simulink library "dspbdsp2"  (Simulink 3.00)
values from neighbouring files (symbols this model uses):
  b = tmp(end-3:end)    [aboutdspblks.m]    (also in dspcsum.m = find_system(blk,'LookUnderMasks','all', 'FollowLinks','on', )
libraries: simulink3 x5, dspbdsp2 x2, dspvect2 x2, dspddes2 x1, dspmtrx2 x1, dsplinalg x1
settings Model: Creator=szlotkin  LastModifiedBy=sconahan

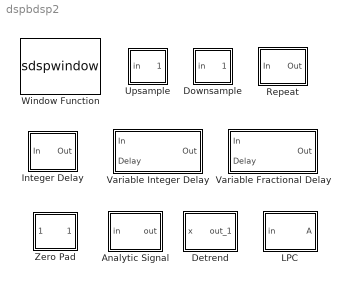
== system dspbdsp2 ==
  Analytic Signal : Subsystem  mask(Analytic Signal){N=100, frame=off, numChans=1}
      mask prompts: N "Filter order (must be even):"; frame "Frame-Based Inputs:"; numChans "Number of Channels"
      mask help: Complex analytic signal of input.
      mask init:
      | [x,y] = dspblkanalytic('icon');
      mask Help: web(dspbhelp);
      mask CallbackString: |dspblkanalytic|
      mask Display: plot(x,y)
  Detrend : Subsystem
      mask Type: Detrend
      mask Description: Remove linear trend from vector input.
      mask Help: web(dspbhelp);
      mask Display: plot(0,0,100,100,[12 20 24 32 38 44 49 54 67 69 71 78 81 89],[56 76 60 79 75 83 80 87 65 76 84 86 91 89],[],[],[],[],[],[],[12 20 24 32 38 44 49 54 67 69 71 78 81 89],[12 31 13 31 27 34 30 36 13 23 30 31 34 32],[4 96],[61 90],[47 47 42 47 52],[64 44 50 44 50],[4 96],[23 23])
  Downsample : Subsystem  mask(Downsample){N=2, phase=0, ic=0, sample_mode=off, frame=off, nchans=1, mode=Maintain input frame size}
      mask prompts: N "Downsample factor, N:"; phase "Sample offset (0 to N-1):"; ic "Initial condition:"; sample_mode "Enforce single-rate"; frame "Frame-based inputs"; nchans "Number of channels:"; mode "Framing:"
      mask help: Downsample by an integer factor. Optional sample offset must be an integer in range (0, N-1).
      mask init:
      | [s,x,y] = dspblkdsamp('icon',N, &1);
      mask Help: web(dspbhelp);
      mask StyleString: edit,edit,edit,checkbox,checkbox,edit,popup(Maintain input frame size|Maintain input frame rate)
      mask CallbackString: ||||dspblkdsamp||
      mask Display:
      | plot(x,y);
      | text(.6,.4,s);
  Integer Delay : Subsystem  mask(Integer Delay){delay=1, ic=0, frame=off, df=on, numChans=1}
      mask prompts: delay "Delay in samples:"; ic "Initial Conditions:"; frame "Frame-Based Inputs"; df "Direct Feedthrough (deselect only if delay >= frame size)"; numChans "Number of Channels:"
      mask help:
      | Delay discrete-time input by a fixed integer number of sample periods.
      |
      | In frame-based mode, feedback loops can be made computable by deselecting "Direct Feedthrough".  This is valid only if the minimum delay value is at least as large as the frame size.
      mask init:
      | str = ['-' &1];
      | dx = 0.01*length(str);
      | if strcmp(frame,'off'), numChans=-1; end
      | delay=double(delay);
      mask Help: web(dspbhelp);
      mask CallbackString: ||dspblkdly||
      mask Display: text(0.42-dx, 0.4, 'z'); text(0.5-dx, 0.6, str);
  LPC : Subsystem  mask(LPC){ord=-1}
      mask prompts: ord "Prediction order (-1 for length(u)-1):"
      mask help: Output the coefficients of an Nth order forward linear predictor such that the sum of the squares of the errors is minimized.
      mask init:
      | if ord==-1,
      |    pad = -1; acf=-1;
      | else
      |    pad = ord+1; acf=ord;
      | end
      mask Help: web(dspbhelp);
      mask Display: disp('LPC')
  Repeat : Subsystem  mask(Repeat){N=5, ic=0, frame=off, nchans=1, mode=Maintain input frame size}
      mask prompts: N "Repetition count:"; ic "Initial conditions:"; frame "Frame-based inputs"; nchans "Number of channels:"; mode "Framing:"
      mask help: Repeat input samples N times.
      mask init:
      | s = dspblkrepeat('icon',N, &1);
      mask Help: web(dspbhelp);
      mask StyleString: edit,edit,checkbox,edit,popup(Maintain input frame size|Maintain input frame rate)
      mask CallbackString: ||dspblkrepeat||
      mask Display: disp(s);
  Upsample : Subsystem  mask(Upsample){N=3, phase=0, ic=0, frame=off, nchans=1, mode=Maintain input frame size}
      mask prompts: N "Upsample factor, N:"; phase "Sample offset (0 to N-1):"; ic "Initial condition:"; frame "Frame-based inputs"; nchans "Number of channels:"; mode "Framing:"
      mask help: Upsample by inserting N-1 zeros between input samples. Optional sample offset must be an integer in range (0, N-1).
      mask init:
      | [s,x,y] = dspblkupsamp('icon',N, &1);
      mask Help: web(dspbhelp);
      mask StyleString: edit,edit,edit,checkbox,edit,popup(Maintain input frame size|Maintain input frame rate)
      mask CallbackString: |||dspblkupsamp||
      mask Display:
      | plot(x,y)
      | text(.6,.4,s);
  Variable Fractional Delay : Subsystem  mask(Variable Fractional Delay){mode=Linear Interpolation, dmax=100, L=4, R=10, alpha=0.5, ic=0, frame=off, numChans=1}
      mask prompts: dmax "Maximum delay in samples:"; L "Interpolation filter half-length:"; R "Interpolation points per input sample:"; alpha "Normalized input bandwidth (0 to 1):"; ic "Initial Conditions:"; frame "Frame-Based Inputs"; numChans "Number of Channels:"
      mask help: Delay discrete-time input by a time-varying fractional number of sample periods, as specified by the "delay" input. Delay must be a real vector signal with one delay value per frame element. The FIR filter is designed using "intfilt" from the Signal Processing Toolbox.
      mask init:
      | [b,str] = dspblkvfdly(mode,R,L,alpha);
      | if strcmp(frame,'off'), numChans=-1; end
      mask Help: web(dspbhelp);
      mask StyleString: popup(Linear Interpolation|FIR Interpolation),edit,edit,edit,edit,edit,checkbox,edit
      mask CallbackString: dspblkvfdly||||||dspblkvfdly|
      mask Display:
      | text(0.5,0.4,'z','horiz','right')
      | text(0.5,0.6,'-f','horiz','left')
  Variable Integer Delay : Subsystem  mask(Variable Integer Delay){dmax=100, ic=0, frame=off, numChans=1}
      mask prompts: dmax "Maximum delay in samples:"; ic "Initial Conditions:"; frame "Frame-Based Inputs"; numChans "Number of Channels:"
      mask help: Delay discrete-time input by a time-varying integer number of sample periods specified by the "delay" input. Delay is a real vector signal with one delay value per sample period. For frame-based operation, the delay input can have one delay per sample period or one delay per frame.
      mask init:
      | str = dspblkvidly(1);
      | if strcmp(frame,'off'), numChans=-1; end
      mask Help: web(dspbhelp);
      mask CallbackString: ||dspblkvidly|
      mask Display:
      | text(0.5,0.4,'z','horiz','right')
      | text(0.5,0.6,'-i','horiz','left')
  Window Function : S-Function  FunctionName=sdspwindow  Parameters=winmode,wintype,N,Rs,beta,winsamp,NChans  PortCounts=[]  SFunctionModules=''  mask(Window Function){winmode=Apply window to input, wintype=Hamming, N=64, Rs=50, beta=10, winsamp=Symmetric, NChans=1}
      mask prompts: winmode "Operation:"; wintype "Window Type:"; N "Window length:"; Rs "Stopband attenuation in dB:"; winsamp "Sampling:"; NChans "Number of channels:"
      mask help: Generate window function and apply to input vector.
      mask init:
      | [x,y,str,ports] = dspblkwinfcn('icon',Rs,beta);
      mask Help: web(dspbhelp);
      mask StyleString: popup(Apply window to input|Generate window|Generate and apply window),popup(Bartlett|Blackman|Boxcar|Chebyshev|Hamming|Hann|Hanning|Kaiser|Triang),edit,edit,edit,popup(Symmetric|Periodic),edit
      mask CallbackString: dspblkwinfcn|dspblkwinfcn|||||
      mask Display:
      | plot(x,y); text(.2,.85,str);
      | port_label(ports(1).type,ports(1).port,ports(1).txt);
      | port_label(ports(2).type,ports(2).port,ports(2).txt);
      | port_label(ports(3).type,ports(3).port,ports(3).txt);
  Zero Pad : Subsystem  mask(Zero Pad){pad=-1, trunc=on, nchans=1}
      mask prompts: pad "Output frame size (-1 to inherit input size):"; trunc "Allow truncation of input"; nchans "Number of channels:"
      mask help: Pad input frame with zeros.
      mask Help: web(dspbhelp);
      mask Display: plot(0,0,100,100,[51 44 44 51],[92 92 8 8],[73 80 80 73],[92 92 8 8],[56 68],[80 80],[56 68],[72 72],[56 68],[64 64],[56 68],[56 56],[56 68],[48 48],[56 68],[40 40],[64 60 56 55 56 60 64 68 69 68 64],[32 32 28 22 16 12 12 16 22 28 32],[24 24 40 36 40 36],[52 24 24 28 24 20])

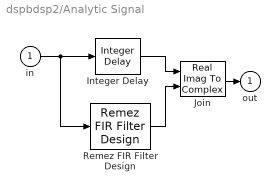
== system dspbdsp2/Analytic Signal ==
  in : Inport  Port=1  PortWidth=-1  SampleTime=-1  DataType=auto
      settings: SignalType=auto
  Integer Delay : dspbdsp2/Integer Delay  delay=N/2  ic=0  frame=off  df=on  numChans=1
  Join : RealImagToComplex  Input=RealAndImag  ConstantPart=0
  Remez FIR Filter Design : dspddes2/Remez FIR Filter Design  filttype=Hilbert Transform  F=[0.05 .95]  A=[1 1]  W=1  N=N  frame=off  numCHANS=1
  out : Outport  Port=1  InitialOutput=0
  wires:
  in/1 -> Remez FIR Filter Design/1, Integer Delay/1
  Join/1 -> out/1
  Integer Delay/1 -> Join/1
  Remez FIR Filter Design/1 -> Join/2

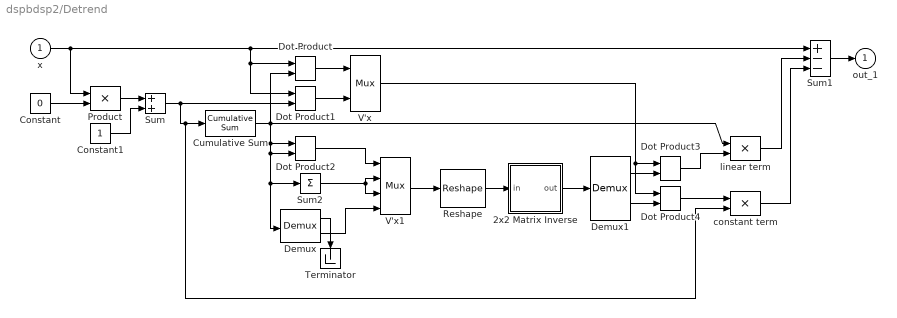
== system dspbdsp2/Detrend ==
  x : Inport  Port=1  PortWidth=-1  SampleTime=-1  DataType=auto
      settings: SignalType=auto
  2x2 Matrix Inverse : Subsystem
      mask Type: Invert 2x2 Matrix
      mask Display: disp('Invert\n2x2')
  Constant : Constant  Value=0
  Constant1 : Constant  Value=1
  Cumulative Sum : dspvect2/Cumulative Sum
  Demux : Demux  Outputs=[-1 1]
  Demux1 : Demux  Outputs=[2 2]
  Dot Product{,1..4} (5 alike) : simulink3/Math/Dot Product
  Product : Product  Inputs=2  SaturateOnIntegerOverflow=on
  Reshape : dspmtrx2/Reshape  Asiz=[2 2]
  Sum : Sum  Inputs=++  SaturateOnIntegerOverflow=on
  Sum1 : Sum  Inputs=+--  SaturateOnIntegerOverflow=on
  Sum2 : Sum  Inputs=+  SaturateOnIntegerOverflow=on
  Terminator : Terminator
      settings: Orientation=down
  V'x : Mux  Inputs=2
      settings: DisplayOption=none
  V'x1 : Mux  Inputs=4
      settings: DisplayOption=none
  constant term : Product  Inputs=2  SaturateOnIntegerOverflow=on
  linear term : Product  Inputs=2  SaturateOnIntegerOverflow=on
  out_1 : Outport  Port=1  InitialOutput=0
  wires:
  V'x/1 -> Dot Product3/1, Dot Product4/1
  x/1 -> Dot Product1/1, Dot Product/1, Sum1/1, Product/1
  Demux1/1 -> Dot Product3/2
  Demux1/2 -> Dot Product4/2
  Dot Product3/1 -> linear term/2
  Dot Product4/1 -> constant term/1
  linear term/1 -> Sum1/2
  constant term/1 -> Sum1/3
  Constant1/1 -> Sum/2
  Product/1 -> Sum/1
  Constant/1 -> Product/2
  Dot Product/1 -> V'x/1
  Dot Product1/1 -> V'x/2
  Sum/1 -> Dot Product1/2, constant term/2, Cumulative Sum/1
  Cumulative Sum/1 -> linear term/1, Dot Product/2, Dot Product2/2, Demux/1, Sum2/1, Dot Product2/1
  Demux/1 -> Terminator/1
  Dot Product2/1 -> V'x1/1
  Demux/2 -> V'x1/4
  Sum2/1 -> V'x1/2, V'x1/3
  Sum1/1 -> out_1/1
  2x2 Matrix Inverse/1(out) -> Demux1/1
  V'x1/1 -> Reshape/1
  Reshape/1 -> 2x2 Matrix Inverse/1(in)

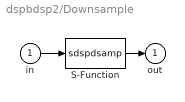
== system dspbdsp2/Downsample ==
  in : Inport  Port=1  PortWidth=-1  SampleTime=-1  DataType=auto
      settings: SignalType=auto
  S-Function : S-Function  FunctionName=sdspdsamp  Parameters=N,phase,ic,sample_mode,frame,nchans,mode  PortCounts=[]  SFunctionModules=''
  out : Outport  Port=1  InitialOutput=0
  wires:
  in/1 -> S-Function/1
  S-Function/1 -> out/1

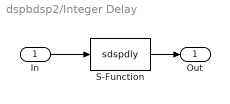
== system dspbdsp2/Integer Delay ==
  In : Inport  Port=1  PortWidth=-1  SampleTime=-1  DataType=auto
      settings: SignalType=auto
  S-Function : S-Function  FunctionName=sdspdly  Parameters=delay,ic,numChans,df  PortCounts=[]  SFunctionModules=''
  Out : Outport  Port=1  InitialOutput=0
  wires:
  S-Function/1 -> Out/1
  In/1 -> S-Function/1

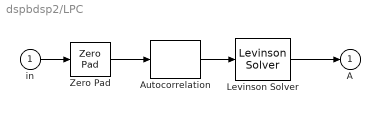
== system dspbdsp2/LPC ==
  in : Inport  Port=1  PortWidth=-1  SampleTime=-1  DataType=auto
      settings: SignalType=auto
  Autocorrelation : dspvect2/Autocorrelation  maxlag=acf  bias=Biased
  Levinson Solver : dsplinalg/Levinson Solver  fcn=A  otype=on
  Zero Pad : dspbdsp2/Zero Pad  pad=pad  trunc=off  nchans=1
  A : Outport  Port=1  InitialOutput=0
  wires:
  in/1 -> Zero Pad/1
  Zero Pad/1 -> Autocorrelation/1
  Levinson Solver/1 -> A/1
  Autocorrelation/1 -> Levinson Solver/1

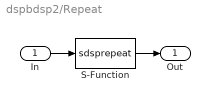
== system dspbdsp2/Repeat ==
  In : Inport  Port=1  PortWidth=-1  SampleTime=-1  DataType=auto
      settings: SignalType=auto
  S-Function : S-Function  FunctionName=sdsprepeat  Parameters=N,ic,frame,nchans,mode  PortCounts=[]  SFunctionModules=''
  Out : Outport  Port=1  InitialOutput=0
  wires:
  S-Function/1 -> Out/1
  In/1 -> S-Function/1

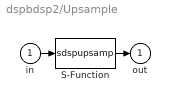
== system dspbdsp2/Upsample ==
  in : Inport  Port=1  PortWidth=-1  SampleTime=-1  DataType=auto
      settings: SignalType=auto
  S-Function : S-Function  FunctionName=sdspupsamp  Parameters=N,phase,ic,frame,nchans,mode  PortCounts=[]  SFunctionModules=''
  out : Outport  Port=1  InitialOutput=0
  wires:
  S-Function/1 -> out/1
  in/1 -> S-Function/1

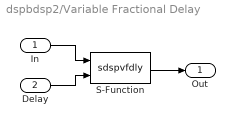
== system dspbdsp2/Variable Fractional Delay ==
  In : Inport  Port=1  PortWidth=-1  SampleTime=-1  DataType=auto
      settings: SignalType=auto
  Delay : Inport  Port=2  PortWidth=-1  SampleTime=-1  DataType=auto
      settings: SignalType=auto
  S-Function : S-Function  FunctionName=sdspvfdly  Parameters=dmax,b,ic,numChans  PortCounts=[]  SFunctionModules=''
  Out : Outport  Port=1  InitialOutput=0
  wires:
  S-Function/1 -> Out/1
  Delay/1 -> S-Function/2
  In/1 -> S-Function/1

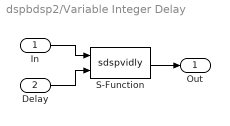
== system dspbdsp2/Variable Integer Delay ==
  In : Inport  Port=1  PortWidth=-1  SampleTime=-1  DataType=auto
      settings: SignalType=auto
  Delay : Inport  Port=2  PortWidth=-1  SampleTime=-1  DataType=auto
      settings: SignalType=auto
  S-Function : S-Function  FunctionName=sdspvidly  Parameters=dmax,ic,numChans  PortCounts=[]  SFunctionModules=''
  Out : Outport  Port=1  InitialOutput=0
  wires:
  S-Function/1 -> Out/1
  In/1 -> S-Function/1
  Delay/1 -> S-Function/2

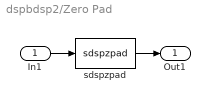
== system dspbdsp2/Zero Pad ==
  In1 : Inport  Port=1  PortWidth=-1  SampleTime=-1  DataType=auto
      settings: SignalType=auto
  sdspzpad : S-Function  FunctionName=sdspzpad  Parameters=pad,trunc,nchans  PortCounts=[]  SFunctionModules=''
  Out1 : Outport  Port=1
  wires:
  sdspzpad/1 -> Out1/1
  In1/1 -> sdspzpad/1

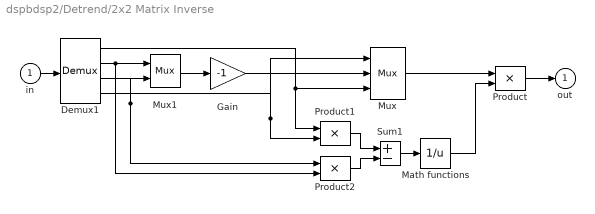
== system dspbdsp2/Detrend/2x2 Matrix Inverse ==
  in : Inport  Port=1  PortWidth=-1  SampleTime=-1  DataType=auto
      settings: SignalType=auto
  Demux1 : Demux  Outputs=4
  Gain : Gain  Gain=-1  SaturateOnIntegerOverflow=on
  Math functions : Math  Operator=reciprocal  OutputSignalType=auto
  Mux : Mux  Inputs=3
      settings: DisplayOption=none
  Mux1 : Mux  Inputs=2
      settings: DisplayOption=none
  Product : Product  Inputs=2  SaturateOnIntegerOverflow=on
  Product1 : Product  Inputs=2  SaturateOnIntegerOverflow=on
  Product2 : Product  Inputs=2  SaturateOnIntegerOverflow=on
  Sum1 : Sum  Inputs=+-  SaturateOnIntegerOverflow=on
  out : Outport  Port=1  InitialOutput=0
  wires:
  Math functions/1 -> Product/2
  Product1/1 -> Sum1/1
  Product2/1 -> Sum1/2
  Sum1/1 -> Math functions/1
  Demux1/4 -> Product1/2, Mux/1
  in/1 -> Demux1/1
  Demux1/1 -> Mux/3, Product1/1
  Demux1/3 -> Product2/1, Mux1/2
  Demux1/2 -> Mux1/1, Product2/2
  Product/1 -> out/1
  Gain/1 -> Mux/2
  Mux1/1 -> Gain/1
  Mux/1 -> Product/1
